simulink model "Nulldynamik"  (R2015b)
settings: Solver=ode15s  StartTime=0.0  StopTime=5  RelTol=1e-3
settings Model: Creator=jens  LastModifiedBy=jens

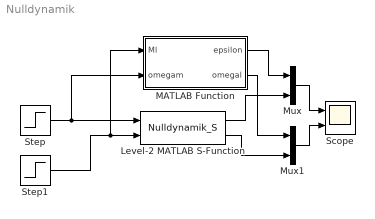
== system Nulldynamik ==
  Level-2 MATLAB S-Function : M-S-Function  FunctionName=Nulldynamik_S  Parameters=parSys
  MATLAB Function : MATLAB Function  TreatAsAtomicUnit=on
  Mux : Mux  Inputs=2
  Mux1 : Mux  Inputs=2
  Scope : Scope  NumInputPorts=2
  Step : Step  Time=0.5  SampleTime=0
  Step1 : Step  Time=1.5  After=50  SampleTime=0
  wires:
  Step/1 -> MATLAB Function/2(omegam), Level-2 MATLAB S-Function/1
  Step1/1 -> MATLAB Function/1(Ml), Level-2 MATLAB S-Function/2
  MATLAB Function/1(epsilon) -> Mux/1
  MATLAB Function/2(omegal) -> Mux1/1
  Level-2 MATLAB S-Function/1 -> Mux/2
  Level-2 MATLAB S-Function/2 -> Mux1/2
  Mux/1 -> Scope/1
  Mux1/1 -> Scope/2

== matlab function Nulldynamik/MATLAB Function ==
  settings: updateMethod=DISCRETE  sampleTime=parSys.TsID
  data: Ml input; omegam input; epsilon output; parSys parameter; omegal output
function [epsilon, omegal] = fcn(Ml,omegam,parSys)
%#codegen

persistent etakm1;
persistent ukm1;

if isempty(etakm1)
    etakm1 = [parSys.eta_1_0 parSys.eta_2_0];
end
if isempty(ukm1)
    ukm1 = [Ml omegam];
end

Il  = parSys.Il;
cr1 = parSys.cr1;
cr3 = parSys.cr3;
dl  = parSys.dl;
rl  = parSys.rl;
Im  = parSys.Im;
dm  = parSys.dm;
rm  = parSys.rm;
Rm  = parSys.Rm;
Lm  = parSys.Lm;
p   = parSys.p;
Phi = parSys.Phi;

Mlk     = Ml;
omegamk = omegam;

epsilon = etakm1(1);
omegal  = etakm1(2);
Ml      = ukm1(1);
omegam  = ukm1(2);

etapkm1 = [omegal * rl - omegam * rm 1 / Il * (-2 * (cr3 * epsilon ^ 3 + cr1 * epsilon) * rl - dl * omegal + Ml)];

etakP = etakm1 + parSys.TsID * etapkm1;

epsilon = etakP(1);
omegal  = etakP(2);
Ml     = Mlk;
omegam = omegamk;

etapP = [omegal * rl - omegam * rm 1 / Il * (-2 * (cr3 * epsilon ^ 3 + cr1 * epsilon) * rl - dl * omegal + Ml)];

etak = etakm1 + parSys.TsID / 2 * (etapkm1 + etapP);

epsilon = etak(1);
omegal  = etak(2);

etakm1 = etak;
ukm1 = [Mlk omegamk];
